simulink model "Encoder_reader_simulink"  (R2025a)
settings: Solver=FixedStepAuto  StartTime=0.0  StopTime=inf  FixedStep=0.001  RelTol=1e-3  EnableMultiTasking=on
libraries: stm32f4xxblockslib x6, stm32g4xxblockslib x4
settings Model: STM32="{\"EncoderBlockForG4\":[{\"ID\":\"untitled:1\"},{\"ID\":\"Lab3_Encoder:1\"},{\"ID\":\"Encoder_reader_simulink:1\"},{\"ID\":\"Encoder_reader_simulink:31\"},{\"ID\":\"Encoder_reader_simulink:37\"},{\"ID\":\"Encoder_reader_simulink:50\"}],\"DigitalPortRead\":[{\"ID\":\"Encoder_reader_simulink:26\"},{\"ID\":\"Encoder_reader_simulink:29\"},{\"ID\":\"Encoder_reader_simulink:35\"},{\"ID\":\"Encoder_reader_simulink:40\"},{\"ID\":\"Encoder_reader_simulink:41\"},{\"ID\":\"Encoder_reader_simulink:48\"}]}"  Creator=User  LastModifiedBy=witch
settings OptimizationCC: DefaultParameterBehavior=Inlined  EnhancedBackFolding=on  PassReuseOutputArgsAs=Individual arguments  ZeroExternalMemoryAtStartup=off  ZeroInternalMemoryAtStartup=off  MaxStackSize=512  OptimizeBlockOrder=speed  DifferentSizesBufferReuse=on  OptimizationCustomize=off  EfficientTunableParamExpr=on
settings DebuggingCC: ParameterTunabilityLossMsg=error
settings HardwareCC: ProdBitPerPointer=32.0  ProdBitPerSizeT=32.0  ProdBitPerPtrDiffT=32.0  ProdLargestAtomicInteger=Long  ProdLargestAtomicFloat=Double  ProdWordSize=32.0  ProdLongLongMode=on  ProdHWDeviceType=ARM Compatible->ARM Cortex-M
settings SFSimCC: MATLABDynamicMemAlloc=off
settings RTWCC: SystemTargetFile=ert.tlc  HardwareBoard=STM32G4xx Based  TemplateMakefile=ert_default_tmf  Toolchain=GNU Tools for ARM Embedded Processors  Description=Embedded Coder
settings CodeAppCC: ForceParamTrailComments=on  IgnoreCustomStorageClasses=off  OperatorAnnotations=on  SimulinkDataObjDesc=on  SFDataObjDesc=on  InsertBlockDesc=on
settings ERTTargetCC: ExtModeTransport=3.0  ExtModeStaticAllocSize=2048.0  TargetLangStandard=C99 (ISO)  CodeReplacementLibrary=ARM Cortex-M  SupportContinuousTime=on

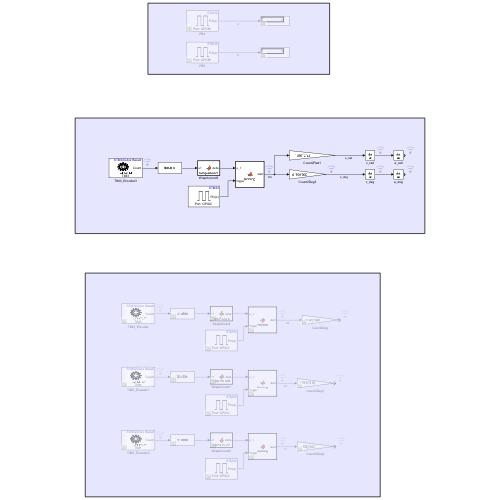
[thumbnail: Simulink's stored preview of the top-level diagram]
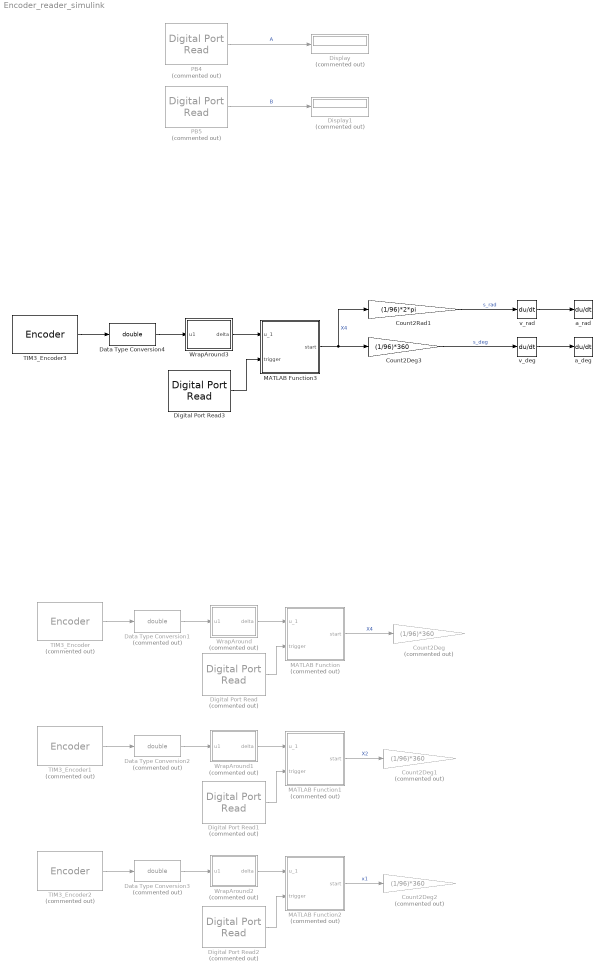
== system Encoder_reader_simulink ==
  Count2Deg : Gain  Commented=on  Gain=(1/96)*360
  Count2Deg1 : Gain  Commented=on  Gain=(1/96)*360
  Count2Deg2 : Gain  Commented=on  Gain=(1/96)*360
  Count2Deg3 : Gain  Gain=(1/96)*360
  Count2Rad1 : Gain  Gain=(1/96)*2*pi
  Data Type Conversion1 : DataTypeConversion  Commented=on  OutDataTypeStr=double  SaturateOnIntegerOverflow=off  RndMeth=Floor
  Data Type Conversion2 : DataTypeConversion  Commented=on  OutDataTypeStr=double  SaturateOnIntegerOverflow=off  RndMeth=Floor
  Data Type Conversion3 : DataTypeConversion  Commented=on  OutDataTypeStr=double  SaturateOnIntegerOverflow=off  RndMeth=Floor
  Data Type Conversion4 : DataTypeConversion  OutDataTypeStr=double  SaturateOnIntegerOverflow=off  RndMeth=Floor
  Digital Port Read : stm32f4xxblockslib/Digital Port Read  Commented=on  PortName=GPIOC  PinNumber=[13]  ReadOperation=on  IOAsArray=on  SampleTime=-1  EnableSimPort=off  hoistedMaskSrc=ECSoC/ECSimCodegen/Digital Port Read
  Digital Port Read1 : stm32f4xxblockslib/Digital Port Read  Commented=on  PortName=GPIOC  PinNumber=[13]  ReadOperation=on  IOAsArray=on  SampleTime=-1  EnableSimPort=off  hoistedMaskSrc=ECSoC/ECSimCodegen/Digital Port Read
  Digital Port Read2 : stm32f4xxblockslib/Digital Port Read  Commented=on  PortName=GPIOC  PinNumber=[13]  ReadOperation=on  IOAsArray=on  SampleTime=-1  EnableSimPort=off  hoistedMaskSrc=ECSoC/ECSimCodegen/Digital Port Read
  Digital Port Read3 : stm32f4xxblockslib/Digital Port Read  PortName=GPIOC  PinNumber=[13]  ReadOperation=on  IOAsArray=on  SampleTime=-1  EnableSimPort=off  hoistedMaskSrc=ECSoC/ECSimCodegen/Digital Port Read
  Display : Display  Commented=on
  Display1 : Display  Commented=on
  MATLAB Function : MATLAB Function  Commented=on  TreatAsAtomicUnit=on
  MATLAB Function1 : MATLAB Function  Commented=on  TreatAsAtomicUnit=on
  MATLAB Function2 : MATLAB Function  Commented=on  TreatAsAtomicUnit=on
  MATLAB Function3 : MATLAB Function  TreatAsAtomicUnit=on
  PB4 : stm32f4xxblockslib/Digital Port Read  Commented=on  PortName=GPIOB  PinNumber=[4]  ReadOperation=on  IOAsArray=on  SampleTime=-1  EnableSimPort=off  hoistedMaskSrc=ECSoC/ECSimCodegen/Digital Port Read
  PB5 : stm32f4xxblockslib/Digital Port Read  Commented=on  PortName=GPIOB  PinNumber=[5]  ReadOperation=on  IOAsArray=on  SampleTime=-1  EnableSimPort=off  hoistedMaskSrc=ECSoC/ECSimCodegen/Digital Port Read
  TIM3_Encoder : stm32g4xxblockslib/Encoder  Commented=on  TimerModule=TIM3  EnableResetInput=off  OutputCountAfterFirstIndex=off  OutputValidIndex=off  OutputDirection=off  OutputStatus=off  SampleTime=-1
  TIM3_Encoder1 : stm32g4xxblockslib/Encoder  Commented=on  TimerModule=TIM4  EnableResetInput=off  OutputCountAfterFirstIndex=off  OutputValidIndex=off  OutputDirection=off  OutputStatus=off  SampleTime=-1
  TIM3_Encoder2 : stm32g4xxblockslib/Encoder  Commented=on  TimerModule=TIM1  EnableResetInput=off  OutputCountAfterFirstIndex=off  OutputValidIndex=off  OutputDirection=off  OutputStatus=off  SampleTime=-1
  TIM3_Encoder3 : stm32g4xxblockslib/Encoder  TimerModule=TIM3  EnableResetInput=off  OutputCountAfterFirstIndex=off  OutputValidIndex=off  OutputDirection=off  OutputStatus=off  SampleTime=-1
  WrapAround : MATLAB Function  Commented=on  TreatAsAtomicUnit=on
  WrapAround1 : MATLAB Function  Commented=on  TreatAsAtomicUnit=on
  WrapAround2 : MATLAB Function  Commented=on  TreatAsAtomicUnit=on
  WrapAround3 : MATLAB Function  TreatAsAtomicUnit=on
  a_deg : Derivative
  a_rad : Derivative
  v_deg : Derivative
  v_rad : Derivative
  wires:
  TIM3_Encoder/1 -> Data Type Conversion1/1
  Data Type Conversion1/1 -> WrapAround/1(u1)
  Count2Rad1/1 -> v_rad/1  "s_rad"
  v_rad/1 -> a_rad/1
  v_deg/1 -> a_deg/1
  WrapAround/1(delta) -> MATLAB Function/1(u_1)
  MATLAB Function/1(start) -> Count2Deg/1  "X4"
  Digital Port Read/1 -> MATLAB Function/2(trigger)
  Digital Port Read1/1 -> MATLAB Function1/2(trigger)
  WrapAround1/1(delta) -> MATLAB Function1/1(u_1)
  Data Type Conversion2/1 -> WrapAround1/1(u1)
  MATLAB Function1/1(start) -> Count2Deg1/1  "X2"
  TIM3_Encoder1/1 -> Data Type Conversion2/1
  Digital Port Read2/1 -> MATLAB Function2/2(trigger)
  MATLAB Function2/1(start) -> Count2Deg2/1  "x1"
  TIM3_Encoder2/1 -> Data Type Conversion3/1
  Data Type Conversion3/1 -> WrapAround2/1(u1)
  WrapAround2/1(delta) -> MATLAB Function2/1(u_1)
  PB4/1 -> Display/1  "A"
  PB5/1 -> Display1/1  "B"
  Digital Port Read3/1 -> MATLAB Function3/2(trigger)
  WrapAround3/1(delta) -> MATLAB Function3/1(u_1)
  Data Type Conversion4/1 -> WrapAround3/1(u1)
  MATLAB Function3/1(start) -> Count2Deg3/1, Count2Rad1/1  "X4"
  TIM3_Encoder3/1 -> Data Type Conversion4/1
  Count2Deg3/1 -> v_deg/1  "s_deg"

== matlab function Encoder_reader_simulink/WrapAround ==
  data: u1 input; delta output
function delta = WrapAround(u1)

    persistent u0
    persistent total_delta
    Counter_Period = 65535;

    if isempty(u0)
        u0 = u1;
    end

    if isempty(total_delta)
        total_delta = 0;
    end

    diff = u1 - u0;

    if diff > Counter_Period/2
        diff = diff - Counter_Period;   
    elseif diff < -Counter_Period/2
        diff = diff + Counter_Period;   
    end

    total_delta = total_delta + diff;
    delta = total_delta;

    u0 = u1;
end

== matlab function Encoder_reader_simulink/MATLAB Function1 ==
  data: u_1 input; start output; trigger input

function start = Homing(u_1, trigger) 

persistent home 

if isempty(home) 
    home = 0; 
end

if trigger 
    home = u_1; 
end

start = u_1 - home;

== matlab function Encoder_reader_simulink/WrapAround1 ==
  data: u1 input; delta output
function delta = WrapAround(u1)

    persistent u0
    persistent total_delta
    Counter_Period = 65535;

    if isempty(u0)
        u0 = u1;
    end

    if isempty(total_delta)
        total_delta = 0;
    end

    diff = u1 - u0;

    if diff > Counter_Period/2
        diff = diff - Counter_Period;   
    elseif diff < -Counter_Period/2
        diff = diff + Counter_Period;   
    end

    total_delta = total_delta + diff;
    delta = total_delta;

    u0 = u1;
end

== matlab function Encoder_reader_simulink/MATLAB Function2 ==
  data: u_1 input; start output; trigger input

function start = Homing(u_1, trigger) 

persistent home 

if isempty(home) 
    home = 0; 
end

if trigger 
    home = u_1; 
end

start = u_1 - home;

== matlab function Encoder_reader_simulink/WrapAround2 ==
  data: u1 input; delta output
function delta = WrapAround(u1)

    persistent u0
    persistent total_delta
    Counter_Period = 65535;

    if isempty(u0)
        u0 = u1;
    end

    if isempty(total_delta)
        total_delta = 0;
    end

    diff = u1 - u0;

    if diff > Counter_Period/2
        diff = diff - Counter_Period;   
    elseif diff < -Counter_Period/2
        diff = diff + Counter_Period;   
    end

    total_delta = total_delta + diff;
    delta = total_delta;

    u0 = u1;
end

== matlab function Encoder_reader_simulink/MATLAB Function3 ==
  data: u_1 input; start output; trigger input

function start = Homing(u_1, trigger) 

persistent home 

if isempty(home) 
    home = 0; 
end

if trigger 
    home = u_1; 
end

start = u_1 - home;

== matlab function Encoder_reader_simulink/WrapAround3 ==
  data: u1 input; delta output
function delta = WrapAround(u1)

    persistent u0
    persistent total_delta
    Counter_Period = 65535;

    if isempty(u0)
        u0 = u1;
    end

    if isempty(total_delta)
        total_delta = 0;
    end

    diff = u1 - u0;

    if diff > Counter_Period/2
        diff = diff - Counter_Period;   
    elseif diff < -Counter_Period/2
        diff = diff + Counter_Period;   
    end

    total_delta = total_delta + diff;
    delta = total_delta;

    u0 = u1;
end

== matlab function Encoder_reader_simulink/MATLAB Function ==
  data: u_1 input; start output; trigger input

function start = Homing(u_1, trigger) 

persistent home 

if isempty(home) 
    home = 0; 
end

if trigger 
    home = u_1; 
end

start = u_1 - home;
